simulink model "dds_cwg_1k"  (R2016b)
(part 11 of 84)

      mask help:
      | An explicitly laid-out delay line to avoid mapping to SRL16s
      | for use in pipelining to help achieve timing closure.
      mask init:
      | pipeline_init(gcb,'latency',latency);
      settings: AttributesFormatString=Latency = %<latency>
      mask Display:
      | port_label('input', 1, 'd');
      | port_label('output', 1, 'q');
      | disp(['Z^-', num2str(latency)]);
  pipeline99 : Subsystem  Commented=on  AncestorBlock=casper_library_delays/pipeline  mask(pipeline){latency=2}
      mask help:
      | An explicitly laid-out delay line to avoid mapping to SRL16s
      | for use in pipelining to help achieve timing closure.
      mask init:
      | pipeline_init(gcb,'latency',latency);
      settings: AttributesFormatString=Latency = %<latency>
      mask Display:
      | port_label('input', 1, 'd');
      | port_label('output', 1, 'q');
      | disp(['Z^-', num2str(latency)]);
  pulse_ext : casper_library_misc/pulse_ext  pulse_len=10
  pulse_ext1 : casper_library_misc/pulse_ext  pulse_len=10
  register_change_detect : Subsystem  Commented=on
  ss_fft : Subsystem  Tag=casper:bitsnap  Commented=on  AncestorBlock=casper_library_scopes/bitfield_snapshot  mask(bitsnap){io_names=[re im ch dv sync of], io_widths=[18 18 15 1 1 1], io_bps=[0 0 0 0 0 0], io_types=[0 0 0 2 2 2], show_format=on, snap_storage=bram, snap_dram_dimm=2, snap_dram_clock=250, snap_nsamples=8, snap_data_width=64, snap_offset=on, snap_circap=off, snap_value=off, snap_ext_arm=off, snap_ext_circ=off, snap_provide_outputs=on, snap_use_dsp48=on, snap_delay=0, extra_names=[c d], extra_widths=[30 2], extra_bps=[0 0], extra_types=0}
      mask prompts: io_names "Names [msb...lsb]"; io_widths "Bitwidths [msb...lsb]"; io_bps "Binary pts [msb...lsb]"; io_types "Data types [msb...lsb], ufix=0, fix=1, bool=2"; show_format "Print format string?"; snap_storage "Storage medium"; snap_dram_dimm "DRAM dimm"; snap_dram_clock "DRAM clock rate"; snap_nsamples "Number of Samples (2^?)"; snap_data_width "Data width"; snap_offset "Start delay support"; snap_circap "Circular capture support"; snap_value "Extra value capture support"; snap_ext_arm "External arm support"; snap_ext_circ "External circular capture support"; snap_provide_outputs "Provide outputs"; snap_use_dsp48 "Use DSP48s to implement counters"; snap_delay "Pre-snapshot delay"; extra_names "Names [msb...lsb]"; extra_widths "Widths [msb...lsb]"; extra_bps "Binary pts [msb...lsb]"; extra_types "Data types [msb...lsb], ufix=0, fix=1, bool=2"
      mask help:
      | A wrapped snapshot block. Allows specification of inputs to a snapblock word so the toolflow can automatically set up the scope.
      | See documentation for snapshot for explanation of parameters.
      mask init:
      | bitsnap_init(gcb);
      settings: AttributesFormatString=|
      | snap(6):uf18.0,uf18.0,uf15.0,b,b,b = 54 bits\n64 wide, 256 deep
      | debugID: 24471511
      mask TypeOptions snap_storage: bram | dram
      mask Callback snap_storage: bitsnap_callback();
      mask TypeOptions snap_dram_dimm: 1 | 2 | 3 | 4
      mask TypeOptions snap_dram_clock: 200 | 250 | 266 | 300 | 333
      mask TypeOptions snap_data_width: 8 | 16 | 32 | 64 | 128
      mask Callback snap_value: bitsnap_callback();
      mask Callback snap_ext_arm: bitsnap_callback();
      mask Callback snap_ext_circ: bitsnap_callback();
      mask Callback snap_provide_outputs: bitsnap_callback();
  ss_fft1 : Subsystem  Tag=casper:bitsnap  Commented=on  AncestorBlock=casper_library_scopes/bitfield_snapshot  mask(bitsnap){io_names=[re im ch dv sync], io_widths=[18 18 15 1 1], io_bps=[0 0 0 0 0], io_types=[0 0 0 2 2], show_format=on, snap_storage=bram, snap_dram_dimm=2, snap_dram_clock=250, snap_nsamples=9, snap_data_width=64, snap_offset=on, snap_circap=off, snap_value=off, snap_ext_arm=off, snap_ext_circ=off, snap_provide_outputs=on, snap_use_dsp48=on, snap_delay=0, extra_names=[c d], extra_widths=[30 2], extra_bps=[0 0], extra_types=0}
      mask prompts: io_names "Names [msb...lsb]"; io_widths "Bitwidths [msb...lsb]"; io_bps "Binary pts [msb...lsb]"; io_types "Data types [msb...lsb], ufix=0, fix=1, bool=2"; show_format "Print format string?"; snap_storage "Storage medium"; snap_dram_dimm "DRAM dimm"; snap_dram_clock "DRAM clock rate"; snap_nsamples "Number of Samples (2^?)"; snap_data_width "Data width"; snap_offset "Start delay support"; snap_circap "Circular capture support"; snap_value "Extra value capture support"; snap_ext_arm "External arm support"; snap_ext_circ "External circular capture support"; snap_provide_outputs "Provide outputs"; snap_use_dsp48 "Use DSP48s to implement counters"; snap_delay "Pre-snapshot delay"; extra_names "Names [msb...lsb]"; extra_widths "Widths [msb...lsb]"; extra_bps "Binary pts [msb...lsb]"; extra_types "Data types [msb...lsb], ufix=0, fix=1, bool=2"
      mask help:
      | A wrapped snapshot block. Allows specification of inputs to a snapblock word so the toolflow can automatically set up the scope.
      | See documentation for snapshot for explanation of parameters.
      mask init:
      | bitsnap_init(gcb);
      settings: AttributesFormatString=|
      | snap(5):uf18.0,uf18.0,uf15.0,b,b = 53 bits\n64 wide, 512 deep
      | debugID: 87522550
      mask TypeOptions snap_storage: bram | dram
      mask Callback snap_storage: bitsnap_callback();
      mask TypeOptions snap_dram_dimm: 1 | 2 | 3 | 4
      mask TypeOptions snap_dram_clock: 200 | 250 | 266 | 300 | 333
      mask TypeOptions snap_data_width: 8 | 16 | 32 | 64 | 128
      mask Callback snap_value: bitsnap_callback();
      mask Callback snap_ext_arm: bitsnap_callback();
      mask Callback snap_ext_circ: bitsnap_callback();
      mask Callback snap_provide_outputs: bitsnap_callback();
  ss_fft2 : Subsystem  Tag=casper:bitsnap  Commented=on  AncestorBlock=casper_library_scopes/bitfield_snapshot  mask(bitsnap){io_names=[re im ch dv sync], io_widths=[18 18 15 1 1], io_bps=[0 0 0 0 0], io_types=[0 0 0 2 2], show_format=on, snap_storage=bram, snap_dram_dimm=2, snap_dram_clock=250, snap_nsamples=9, snap_data_width=64, snap_offset=on, snap_circap=off, snap_value=off, snap_ext_arm=off, snap_ext_circ=off, snap_provide_outputs=on, snap_use_dsp48=on, snap_delay=0, extra_names=[c d], extra_widths=[30 2], extra_bps=[0 0], extra_types=0}
      mask prompts: io_names "Names [msb...lsb]"; io_widths "Bitwidths [msb...lsb]"; io_bps "Binary pts [msb...lsb]"; io_types "Data types [msb...lsb], ufix=0, fix=1, bool=2"; show_format "Print format string?"; snap_storage "Storage medium"; snap_dram_dimm "DRAM dimm"; snap_dram_clock "DRAM clock rate"; snap_nsamples "Number of Samples (2^?)"; snap_data_width "Data width"; snap_offset "Start delay support"; snap_circap "Circular capture support"; snap_value "Extra value capture support"; snap_ext_arm "External arm support"; snap_ext_circ "External circular capture support"; snap_provide_outputs "Provide outputs"; snap_use_dsp48 "Use DSP48s to implement counters"; snap_delay "Pre-snapshot delay"; extra_names "Names [msb...lsb]"; extra_widths "Widths [msb...lsb]"; extra_bps "Binary pts [msb...lsb]"; extra_types "Data types [msb...lsb], ufix=0, fix=1, bool=2"
      mask help:
      | A wrapped snapshot block. Allows specification of inputs to a snapblock word so the toolflow can automatically set up the scope.
      | See documentation for snapshot for explanation of parameters.
      mask init:
      | bitsnap_init(gcb);
      settings: AttributesFormatString=|
      | snap(5):uf18.0,uf18.0,uf15.0,b,b = 53 bits\n64 wide, 512 deep
      | debugID: 87552341
      mask TypeOptions snap_storage: bram | dram
      mask Callback snap_storage: bitsnap_callback();
      mask TypeOptions snap_dram_dimm: 1 | 2 | 3 | 4
      mask TypeOptions snap_dram_clock: 200 | 250 | 266 | 300 | 333
      mask TypeOptions snap_data_width: 8 | 16 | 32 | 64 | 128
      mask Callback snap_value: bitsnap_callback();
      mask Callback snap_ext_arm: bitsnap_callback();
      mask Callback snap_ext_circ: bitsnap_callback();
      mask Callback snap_provide_outputs: bitsnap_callback();
  ss_fft3 : Subsystem  Tag=casper:bitsnap  Commented=on  AncestorBlock=casper_library_scopes/bitfield_snapshot  mask(bitsnap){io_names=[re im shift dv_in sync rst tlast dv_out ch0 re_ou sync_out dvu trdy err fifo], io_widths=[18 18 16 1 1 1 1 1 15 18 1 1 1 1 1], io_bps=[0 0 0 0 0 0 0 0 0 0 0 0 0 0 0], io_types=[0 0 0 2 2 2 2 2 0 0 2 2 2 2 2], show_format=on, snap_storage=bram, snap_dram_dimm=2, snap_dram_clock=250, snap_nsamples=10, snap_data_width=128, snap_offset=on, snap_circap=off, snap_value=off, snap_ext_arm=off, snap_ext_circ=off, snap_provide_outputs=on, snap_use_dsp48=on, snap_delay=0, extra_names=[c d], extra_widths=[30 2], extra_bps=[0 0], extra_types=0}
      mask prompts: io_names "Names [msb...lsb]"; io_widths "Bitwidths [msb...lsb]"; io_bps "Binary pts [msb...lsb]"; io_types "Data types [msb...lsb], ufix=0, fix=1, bool=2"; show_format "Print format string?"; snap_storage "Storage medium"; snap_dram_dimm "DRAM dimm"; snap_dram_clock "DRAM clock rate"; snap_nsamples "Number of Samples (2^?)"; snap_data_width "Data width"; snap_offset "Start delay support"; snap_circap "Circular capture support"; snap_value "Extra value capture support"; snap_ext_arm "External arm support"; snap_ext_circ "External circular capture support"; snap_provide_outputs "Provide outputs"; snap_use_dsp48 "Use DSP48s to implement counters"; snap_delay "Pre-snapshot delay"; extra_names "Names [msb...lsb]"; extra_widths "Widths [msb...lsb]"; extra_bps "Binary pts [msb...lsb]"; extra_types "Data types [msb...lsb], ufix=0, fix=1, bool=2"
      mask help:
      | A wrapped snapshot block. Allows specification of inputs to a snapblock word so the toolflow can automatically set up the scope.
      | See documentation for snapshot for explanation of parameters.
      mask init:
      | bitsnap_init(gcb);
      settings: AttributesFormatString=|
      | snap(15):uf18.0,uf18.0,uf16.0,b,b,b,b,b,uf15.0,uf18.0,b,b,b,b,b = 95 bits\n128 wide, 1024 deep
      | debugID: 87582132
      mask TypeOptions snap_storage: bram | dram
      mask Callback snap_storage: bitsnap_callback();
      mask TypeOptions snap_dram_dimm: 1 | 2 | 3 | 4
      mask TypeOptions snap_dram_clock: 200 | 250 | 266 | 300 | 333
      mask TypeOptions snap_data_width: 8 | 16 | 32 | 64 | 128
      mask Callback snap_value: bitsnap_callback();
      mask Callback snap_ext_arm: bitsnap_callback();
      mask Callback snap_ext_circ: bitsnap_callback();
      mask Callback snap_provide_outputs: bitsnap_callback();
  ss_fft4 : Subsystem  Tag=casper:bitsnap  Commented=on  AncestorBlock=casper_library_scopes/bitfield_snapshot  mask(bitsnap){io_names=[re_i re_o dv we rd sync empty full dv_in dcount], io_widths=[18 18 1 1 1 1 1 1 1 6], io_bps=[0 0 0 0 0 0 0 0 0 0], io_types=[0 0 2 2 2 2 2 2 2 0], show_format=on, snap_storage=bram, snap_dram_dimm=2, snap_dram_clock=250, snap_nsamples=10, snap_data_width=64, snap_offset=on, snap_circap=off, snap_value=off, snap_ext_arm=off, snap_ext_circ=off, snap_provide_outputs=on, snap_use_dsp48=on, snap_delay=0, extra_names=[c d], extra_widths=[30 2], extra_bps=[0 0], extra_types=0}
      mask prompts: io_names "Names [msb...lsb]"; io_widths "Bitwidths [msb...lsb]"; io_bps "Binary pts [msb...lsb]"; io_types "Data types [msb...lsb], ufix=0, fix=1, bool=2"; show_format "Print format string?"; snap_storage "Storage medium"; snap_dram_dimm "DRAM dimm"; snap_dram_clock "DRAM clock rate"; snap_nsamples "Number of Samples (2^?)"; snap_data_width "Data width"; snap_offset "Start delay support"; snap_circap "Circular capture support"; snap_value "Extra value capture support"; snap_ext_arm "External arm support"; snap_ext_circ "External circular capture support"; snap_provide_outputs "Provide outputs"; snap_use_dsp48 "Use DSP48s to implement counters"; snap_delay "Pre-snapshot delay"; extra_names "Names [msb...lsb]"; extra_widths "Widths [msb...lsb]"; extra_bps "Binary pts [msb...lsb]"; extra_types "Data types [msb...lsb], ufix=0, fix=1, bool=2"
      mask help:
      | A wrapped snapshot block. Allows specification of inputs to a snapblock word so the toolflow can automatically set up the scope.
      | See documentation for snapshot for explanation of parameters.
      mask init:
      | bitsnap_init(gcb);
      settings: AttributesFormatString=|
      | snap(10):uf18.0,uf18.0,b,b,b,b,b,b,b,uf6.0 = 49 bits\n64 wide, 1024 deep
      | debugID: 87611923
      mask TypeOptions snap_storage: bram | dram
      mask Callback snap_storage: bitsnap_callback();
      mask TypeOptions snap_dram_dimm: 1 | 2 | 3 | 4
      mask TypeOptions snap_dram_clock: 200 | 250 | 266 | 300 | 333
      mask TypeOptions snap_data_width: 8 | 16 | 32 | 64 | 128
      mask Callback snap_value: bitsnap_callback();
      mask Callback snap_ext_arm: bitsnap_callback();
      mask Callback snap_ext_circ: bitsnap_callback();
      mask Callback snap_provide_outputs: bitsnap_callback();
  ss_fifo_db : Subsystem  Tag=casper:bitsnap  Commented=on  AncestorBlock=casper_library_scopes/bitfield_snapshot  mask(bitsnap){io_names=[din we re rst dout empty full dcount], io_widths=[10 1 1 1 10 1 1 5], io_bps=[0 0 0 0 0 0 0 0], io_types=[0 2 2 2 0 2 2 0], show_format=on, snap_storage=bram, snap_dram_dimm=2, snap_dram_clock=250, snap_nsamples=8, snap_data_width=32, snap_offset=on, snap_circap=off, snap_value=off, snap_ext_arm=off, snap_ext_circ=off, snap_provide_outputs=on, snap_use_dsp48=on, snap_delay=0, extra_names=[c d], extra_widths=[30 2], extra_bps=[0 0], extra_types=0}
      mask prompts: io_names "Names [msb...lsb]"; io_widths "Bitwidths [msb...lsb]"; io_bps "Binary pts [msb...lsb]"; io_types "Data types [msb...lsb], ufix=0, fix=1, bool=2"; show_format "Print format string?"; snap_storage "Storage medium"; snap_dram_dimm "DRAM dimm"; snap_dram_clock "DRAM clock rate"; snap_nsamples "Number of Samples (2^?)"; snap_data_width "Data width"; snap_offset "Start delay support"; snap_circap "Circular capture support"; snap_value "Extra value capture support"; snap_ext_arm "External arm support"; snap_ext_circ "External circular capture support"; snap_provide_outputs "Provide outputs"; snap_use_dsp48 "Use DSP48s to implement counters"; snap_delay "Pre-snapshot delay"; extra_names "Names [msb...lsb]"; extra_widths "Widths [msb...lsb]"; extra_bps "Binary pts [msb...lsb]"; extra_types "Data types [msb...lsb], ufix=0, fix=1, bool=2"
      mask help:
      | A wrapped snapshot block. Allows specification of inputs to a snapblock word so the toolflow can automatically set up the scope.
      | See documentation for snapshot for explanation of parameters.
      mask init:
      | bitsnap_init(gcb);
      settings: AttributesFormatString=|
      | snap(8):uf10.0,b,b,b,uf10.0,b,b,uf5.0 = 30 bits\n32 wide, 256 deep
      | debugID: 59001754
      mask TypeOptions snap_storage: bram | dram
      mask Callback snap_storage: bitsnap_callback();
      mask TypeOptions snap_dram_dimm: 1 | 2 | 3 | 4
      mask TypeOptions snap_dram_clock: 200 | 250 | 266 | 300 | 333
      mask TypeOptions snap_data_width: 8 | 16 | 32 | 64 | 128
      mask Callback snap_value: bitsnap_callback();
      mask Callback snap_ext_arm: bitsnap_callback();
      mask Callback snap_ext_circ: bitsnap_callback();
      mask Callback snap_provide_outputs: bitsnap_callback();
  ss_fir_out : Subsystem  Tag=casper:bitsnap  Commented=on  AncestorBlock=casper_library_scopes/bitfield_snapshot  mask(bitsnap){io_names=[fir_re fir_im dv sync], io_widths=[18 18 1 1], io_bps=[0 17 0 0], io_types=[0 1 2 2], show_format=on, snap_storage=bram, snap_dram_dimm=2, snap_dram_clock=250, snap_nsamples=9, snap_data_width=64, snap_offset=on, snap_circap=off, snap_value=off, snap_ext_arm=off, snap_ext_circ=off, snap_provide_outputs=on, snap_use_dsp48=on, snap_delay=0, extra_names=[c d], extra_widths=[30 2], extra_bps=[0 0], extra_types=0}
      mask prompts: io_names "Names [msb...lsb]"; io_widths "Bitwidths [msb...lsb]"; io_bps "Binary pts [msb...lsb]"; io_types "Data types [msb...lsb], ufix=0, fix=1, bool=2"; show_format "Print format string?"; snap_storage "Storage medium"; snap_dram_dimm "DRAM dimm"; snap_dram_clock "DRAM clock rate"; snap_nsamples "Number of Samples (2^?)"; snap_data_width "Data width"; snap_offset "Start delay support"; snap_circap "Circular capture support"; snap_value "Extra value capture support"; snap_ext_arm "External arm support"; snap_ext_circ "External circular capture support"; snap_provide_outputs "Provide outputs"; snap_use_dsp48 "Use DSP48s to implement counters"; snap_delay "Pre-snapshot delay"; extra_names "Names [msb...lsb]"; extra_widths "Widths [msb...lsb]"; extra_bps "Binary pts [msb...lsb]"; extra_types "Data types [msb...lsb], ufix=0, fix=1, bool=2"
      mask help:
      | A wrapped snapshot block. Allows specification of inputs to a snapblock word so the toolflow can automatically set up the scope.
      | See documentation for snapshot for explanation of parameters.
      mask init:
      | bitsnap_init(gcb);
      settings: AttributesFormatString=|
      | snap(4):uf18.0,f18.17,b,b = 38 bits\n64 wide, 512 deep
      | debugID: 133429805
      mask TypeOptions snap_storage: bram | dram
      mask Callback snap_storage: bitsnap_callback();
      mask TypeOptions snap_dram_dimm: 1 | 2 | 3 | 4
      mask TypeOptions snap_dram_clock: 200 | 250 | 266 | 300 | 333
      mask TypeOptions snap_data_width: 8 | 16 | 32 | 64 | 128
      mask Callback snap_value: bitsnap_callback();
      mask Callback snap_ext_arm: bitsnap_callback();
      mask Callback snap_ext_circ: bitsnap_callback();
      mask Callback snap_provide_outputs: bitsnap_callback();
  ss_nb : Subsystem  Tag=casper:bitsnap  Commented=on  AncestorBlock=casper_library_scopes/bitfield_snapshot  mask(bitsnap){io_names=[r0 i0 r1 i1 sync dv sync_cnt new_spec trig ch], io_widths=[18 18 18 18 1 1 4 1 1 15], io_bps=[17 17 17 17 0 0 0 0 0 0], io_types=[1 1 1 1 2 2 0 2 2 0], show_format=on, snap_storage=bram, snap_dram_dimm=2, snap_dram_clock=250, snap_nsamples=9, snap_data_width=128, snap_offset=off, snap_circap=off, snap_value=off, snap_ext_arm=off, snap_ext_circ=off, snap_provide_outputs=on, snap_use_dsp48=on, snap_delay=2, extra_names=timestamp, extra_widths=32, extra_bps=0, extra_types=0}
      mask prompts: io_names "Names [msb...lsb]"; io_widths "Bitwidths [msb...lsb]"; io_bps "Binary pts [msb...lsb]"; io_types "Data types [msb...lsb], ufix=0, fix=1, bool=2"; show_format "Print format string?"; snap_storage "Storage medium"; snap_dram_dimm "DRAM dimm"; snap_dram_clock "DRAM clock rate"; snap_nsamples "Number of Samples (2^?)"; snap_data_width "Data width"; snap_offset "Start delay support"; snap_circap "Circular capture support"; snap_value "Extra value capture support"; snap_ext_arm "External arm support"; snap_ext_circ "External circular capture support"; snap_provide_outputs "Provide outputs"; snap_use_dsp48 "Use DSP48s to implement counters"; snap_delay "Pre-snapshot delay"; extra_names "Names [msb...lsb]"; extra_widths "Widths [msb...lsb]"; extra_bps "Binary pts [msb...lsb]"; extra_types "Data types [msb...lsb], ufix=0, fix=1, bool=2"
      mask help:
      | A wrapped snapshot block. Allows specification of inputs to a snapblock word so the toolflow can automatically set up the scope.
      | See documentation for snapshot for explanation of parameters.
      mask init:
      | bitsnap_init(gcb);
      settings: AttributesFormatString=|
      | snap(10):f18.17,f18.17,f18.17,f18.17,b,b,uf4.0,b,b,uf15.0 = 95 bits\n128 wide, 512 deep
      | debugID: 12323807
      mask TypeOptions snap_storage: bram | dram
      mask Callback snap_storage: bitsnap_callback();
      mask TypeOptions snap_dram_dimm: 1 | 2 | 3 | 4
      mask TypeOptions snap_dram_clock: 200 | 250 | 266 | 300 | 333
      mask TypeOptions snap_data_width: 8 | 16 | 32 | 64 | 128
      mask Callback snap_value: bitsnap_callback();
      mask Callback snap_ext_arm: bitsnap_callback();
      mask Callback snap_ext_circ: bitsnap_callback();
      mask Callback snap_provide_outputs: bitsnap_callback();
  ss_nb1 : Subsystem  Tag=casper:bitsnap  Commented=on  AncestorBlock=casper_library_scopes/bitfield_snapshot  mask(bitsnap){io_names=[r2 i2 r3 i3 sync dv sync_cnt trig trig_time], io_widths=[18 18 18 18 1 1 4 1 48], io_bps=[17 17 17 17 0 0 0 0 0], io_types=[1 1 1 1 2 2 0 2 0], show_format=on, snap_storage=bram, snap_dram_dimm=2, snap_dram_clock=250, snap_nsamples=9, snap_data_width=128, snap_offset=off, snap_circap=off, snap_value=off, snap_ext_arm=off, snap_ext_circ=off, snap_provide_outputs=on, snap_use_dsp48=on, snap_delay=2, extra_names=timestamp, extra_widths=32, extra_bps=0, extra_types=0}
      mask prompts: io_names "Names [msb...lsb]"; io_widths "Bitwidths [msb...lsb]"; io_bps "Binary pts [msb...lsb]"; io_types "Data types [msb...lsb], ufix=0, fix=1, bool=2"; show_format "Print format string?"; snap_storage "Storage medium"; snap_dram_dimm "DRAM dimm"; snap_dram_clock "DRAM clock rate"; snap_nsamples "Number of Samples (2^?)"; snap_data_width "Data width"; snap_offset "Start delay support"; snap_circap "Circular capture support"; snap_value "Extra value capture support"; snap_ext_arm "External arm support"; snap_ext_circ "External circular capture support"; snap_provide_outputs "Provide outputs"; snap_use_dsp48 "Use DSP48s to implement counters"; snap_delay "Pre-snapshot delay"; extra_names "Names [msb...lsb]"; extra_widths "Widths [msb...lsb]"; extra_bps "Binary pts [msb...lsb]"; extra_types "Data types [msb...lsb], ufix=0, fix=1, bool=2"
      mask help:
      | A wrapped snapshot block. Allows specification of inputs to a snapblock word so the toolflow can automatically set up the scope.
      | See documentation for snapshot for explanation of parameters.
      mask init:
      | bitsnap_init(gcb);
      settings: AttributesFormatString=|
      | snap(9):f18.17,f18.17,f18.17,f18.17,b,b,uf4.0,b,uf48.0 = 127 bits\n128 wide, 512 deep
      | debugID: 113596910
      mask TypeOptions snap_storage: bram | dram
      mask Callback snap_storage: bitsnap_callback();
      mask TypeOptions snap_dram_dimm: 1 | 2 | 3 | 4
      mask TypeOptions snap_dram_clock: 200 | 250 | 266 | 300 | 333
      mask TypeOptions snap_data_width: 8 | 16 | 32 | 64 | 128
      mask Callback snap_value: bitsnap_callback();
      mask Callback snap_ext_arm: bitsnap_callback();
      mask Callback snap_ext_circ: bitsnap_callback();
      mask Callback snap_provide_outputs: bitsnap_callback();
  ss_time_trig_nb : Subsystem  Commented=on
  sync_out : Outport
  dv_out : Outport  Port=2
  pol0_out : Outport  Port=3
  pol1_out : Outport  Port=4
  pfb_of : Outport  Port=5
  tag scope: capture_now=global, current_channel=global, data_pol0=global, fft_ch0=global, fft_ch1=global, fft_conf_tready_p0=global, fft_dv0=global, fft_dv1=global, fft_dvalid=global, fft_p0_fifo_full=global, fft_pol0_err=global, fft_pol0_of=global, fft_pol1_err=global, fft_pol1_of=global, fft_sync0=global, fft_sync=global, fft_sync_count=global, fft_tready_p0=global, fir_data_tlast=global, fir_dvalid_pol0=global, fir_pol0=global, fir_sync=global, reord_channel=global, reord_dv=global, reord_mux_sel=global, reord_pol0=global, reord_pol1=global, reord_sync=global
  wires:
  pfb_fir_generic0/2(pol0_out0) -> pipeline18/1(d)
  pfb_fir_generic1/2(pol0_out0) -> pipeline20/1(d)
  pfb_fir_generic0/1(sync_out) -> pipeline17/1(d)
  pfb_fir_generic1/1(sync_out) -> Terminator5/1
  Reinterpret2/1 -> Concat3/1
  Reinterpret3/1 -> Concat3/2
  Concat3/1 -> [data_pol1]
  pol1/1 -> pfb_fir_generic1/2(pol0_in0)
  Gateway Out21/1 -> To Workspace21/1
  bus_expand1/1(msb_out8) -> Gateway Out21/1
  Gateway Out23/1 -> To Workspace23/1
  bus_expand1/2(out7) -> Gateway Out23/1
  Gateway Out24/1 -> To Workspace24/1
  bus_expand1/3(out6) -> Gateway Out24/1
  Gateway Out25/1 -> To Workspace27/1
  bus_expand1/4(out5) -> Gateway Out25/1
  Gateway Out28/1 -> To Workspace25/1
  bus_expand1/5(out4) -> Gateway Out28/1
  Gateway Out29/1 -> To Workspace28/1
  bus_expand1/6(out3) -> Gateway Out29/1
  Gateway Out30/1 -> To Workspace26/1
  bus_expand1/7(out2) -> Gateway Out30/1
  Gateway Out31/1 -> To Workspace29/1
  bus_expand1/8(lsb_out1) -> Gateway Out31/1
  Gateway Out6/1 -> To Workspace6/1
  Gateway Out1/1 -> To Workspace1/1
  Gateway Out9/1 -> To Workspace9/1
  Gateway Out36/1 -> To Workspace36/1
  Gateway Out39/1 -> To Workspace39/1
  [fft_im_pol1] -> Reinterpret3/1
  [fft_re_pol1] -> Reinterpret2/1
  pfb_fir_generic0/3(dvalid) -> pipeline19/1(d)
  pfb_fir_generic1/3(dvalid) -> pipeline21/1(d)
  Counter1/1 -> pipeline81/1(d), pipeline69/1(d)
  pipeline67/1(q) -> ss_nb/5(in_sync)
  pipeline68/1(q) -> ss_nb/6(in_dv)
  pipeline69/1(q) -> ss_nb/7(in_sync_cnt)
  pipeline70/1(q) -> ss_nb/9(in_trig)
  sync/1 -> pfb_fir_generic1/1(sync), pfb_fir_generic0/1(sync), Gateway Out9/1
  Counter3/1 -> Relational4/1, Gateway Out53/1
  Constant9/1 -> Relational4/2
  bus_expand2/1(msb_out8) -> pipeline87/1(d)
  bus_expand2/2(out7) -> pipeline86/1(d)
  bus_expand2/3(out6) -> pipeline85/1(d)
  bus_expand2/4(out5) -> pipeline84/1(d)
  pipeline84/1(q) -> ss_nb/4(in_i1)
  pipeline85/1(q) -> ss_nb/3(in_r1)
  pipeline86/1(q) -> ss_nb/2(in_i0)
  pipeline87/1(q) -> ss_nb/1(in_r0)
  pipeline79/1(q) -> ss_nb1/5(in_sync)
  pipeline80/1(q) -> ss_nb1/6(in_dv)
  pipeline81/1(q) -> ss_nb1/7(in_sync_cnt)
  pipeline82/1(q) -> ss_nb1/8(in_trig)
  pipeline38/1(q) -> ss_nb1/9(in_trig_time)
  bus_expand2/5(out4) -> pipeline91/1(d)
  bus_expand2/6(out3) -> pipeline90/1(d)
  bus_expand2/7(out2) -> pipeline89/1(d)
  bus_expand2/8(lsb_out1) -> pipeline88/1(d)
  dvalid/1 -> pfb_fir_generic1/3(en), pfb_fir_generic0/3(en), Gateway Out36/1
  Gateway Out70/1 -> To Workspace69/1
  Gateway Out71/1 -> To Workspace70/1
  [fft_re_pol0] -> Gateway Out70/1
  [fft_im_pol0] -> Gateway Out71/1
  pol0/1 -> bus_expand14/1(bus_in), pfb_fir_generic0/2(pol0_in0)
  pipeline88/1(q) -> ss_nb1/4(in_i3)
  pipeline89/1(q) -> ss_nb1/3(in_r3)
  pipeline90/1(q) -> ss_nb1/2(in_i2)
  pipeline91/1(q) -> ss_nb1/1(in_r2)
  pipeline42/1(q) -> ss_nb/8(in_new_spec)
  From149/1 -> pipeline42/1(d)
  fft_shift/1 -> [fft_shift]
  Constant2/1 -> Mux3/2
  [fft_dv0] -> Mux3/1
  Mux3/1 -> [fft_re_pol0]
  Constant1/1 -> Mux4/2
  Mux4/1 -> [fft_im_pol0]
  [fft_re_pol0_int] -> Mux3/3
  [fft_im_pol0_int] -> Mux4/3
  [fft_dv0] -> Mux4/1
  pipeline19/1(q) -> [fir_dvalid_pol0], Gateway Out1/1, Counter3/2
  pipeline20/1(q) -> [fir_pol1]
  pipeline21/1(q) -> [fir_dvalid_pol1]
  pipeline18/1(q) -> [fir_pol0]
  From17/1 -> pipeline79/1(d), pipeline67/1(d)
  [cnt_rst] -> pipeline230/1(d)
  Counter12/1 -> fir_sync_cnt/1(out_reg)
  pipeline229/1(q) -> Counter12/2
  pipeline230/1(q) -> Counter12/1
  From90/1 -> Mux6/1
  Mux6/1 -> edge_detect6/1(in)
  From94/1 -> ss_time_trig_nb/2(rst)
  From91/1 -> ss_time_trig_nb/3(arm)
  ss_time_trig_nb/1(trig) -> Mux6/3
  From95/1 -> ss_time_trig_nb/4(trig_time_in)
  From_pfb_d2/1 -> ss_time_trig_nb/1(current_time)
  From96/1 -> Mux6/2
  pipeline28/1(q) -> ss_nb1/10(we)
  pipeline37/1(q) -> ss_nb/11(we)
  ss_time_trig_nb/2(trig_time) -> pipeline38/1(d)
  edge_detect6/1(out) -> pipeline41/1(d), pipeline82/1(d), pipeline40/1(d), pipeline70/1(d)
  Fast Fourier Transform 9.0 1/1 -> pipeline23/1(d)
  pipeline117/1(q) -> [fft_tready_p0]
  pipeline110/1(q) -> [fft_ch0]
  Gateway Out66/1 -> To Workspace65/1
  Gateway Out67/1 -> To Workspace66/1
  Gateway Out72/1 -> To Workspace71/1
  [fft_dv0] -> Gateway Out67/1
  [fft_ch0] -> Gateway Out66/1
  [fft_tready_p0] -> Gateway Out72/1
  Fast Fourier Transform 9.0 1/5 -> pipeline122/1(d)
  Fast Fourier Transform 9.0 1/6 -> pipeline123/1(d)
  Fast Fourier Transform 9.0 1/8 -> pipeline110/1(d), Relational2/1
  Fast Fourier Transform 9.0 1/15 -> Terminator7/1
  Fast Fourier Transform 9.0 1/16 -> Terminator8/1
  Fast Fourier Transform 9.0 1/17 -> Terminator9/1
  pipeline123/1(q) -> [fft_re_pol0_int]
  pipeline122/1(q) -> [fft_im_pol0_int]
  Inverter1/1 -> Gateway Out41/1, Logical9/2, pipeline62/1(d), Fast Fourier Transform 9.0 1/10
  Gateway Out37/1 -> To Workspace37/1
  [fir_sync] -> pulse_ext/1, Delay9/1
  [fft_sync0] -> Gateway Out37/1
  Concat/1 -> [data_pol0]
  Gateway Out34/1 -> To Workspace32/1
  [fft_sync0] -> [fft_sync]
  [current_channel] -> Gateway Out34/1
  [fft_ch0] -> [current_channel]
  [fft_im_pol0] -> Reinterpret1/1
  [fft_re_pol0] -> Reinterpret/1
  [data_pol0] -> bus_expand16/1(bus_in)
  Gateway Out2/1 -> To Workspace2/1
  Gateway Out5/1 -> To Workspace5/1
  [fft_dv0] -> [fft_dvalid]
  [cnt_rst] -> pipeline27/1(d)
  Counter4/1 -> [fft_sync_count], fft_sync_cnt/1(out_reg)
  pipeline1/1(q) -> Counter4/2
  pipeline27/1(q) -> Counter4/1
  [fft_sync] -> pipeline1/1(d)
  From112/1 -> pipeline68/1(d), pipeline28/1(d), pipeline80/1(d), pipeline37/1(d)
  From114/1 -> bus_expand1/1(bus_in), bus_expand2/1(bus_in)
  Gateway Out18/1 -> To Workspace19/1
  Register11/1 -> Delay26/1
  Register10/1 -> Delay25/1
  Register9/1 -> Delay23/1
  Register1/1 -> Delay22/1
  [capture_now] -> Register1/3
  [capture_now] -> Register9/3
  [capture_now] -> Register10/3
  [capture_now] -> Register11/3
  Gateway Out7/1 -> To Workspace7/1
  Delay19/1 -> Register9/1
  Delay20/1 -> Register10/1
  Gateway Out40/1 -> To Workspace40/1
  [reord_channel] -> Delay5/1
  lsb_1/1 -> Logical4/2
  lsb_0/1 -> Logical4/1
  Logical4/1 -> edge_detect2/1(in)
  [reord_dv] -> Delay1/1
  edge_detect2/1(out) -> [capture_now], Gateway Out40/1
  [capture_now] -> Delay10/1
  Delay10/1 -> Gateway Out61/1, Delay32/1
  Delay1/1 -> Logical4/3
  bus_expand5/1(msb_out2) -> Gateway Out46/1
  bus_expand5/2(lsb_out1) -> Gateway Out49/1
  Delay16/1 -> bus_expand5/1(bus_in), Register1/1
  Gateway Out12/1 -> To Workspace12/1
  Gateway Out13/1 -> To Workspace13/1
  bus_expand4/1(msb_out2) -> Gateway Out13/1
  Gateway Out14/1 -> To Workspace14/1
  bus_expand4/2(lsb_out1) -> Gateway Out14/1
  Gateway Out46/1 -> To Workspace45/1
  Gateway Out49/1 -> To Workspace46/1
  Gateway Out61/1 -> To Workspace49/1
  [reord_dv] -> Delay73/1
  Delay5/1 -> Gateway Out11/1, Delay33/1, Gateway Out12/1, lsb_1/1, lsb_0/1
  Delay33/1 -> Delay34/1
  Gateway Out83/1 -> To Workspace85/1
  [reord_sync] -> Delay78/1
  [reord_pol0] -> Delay74/1
  Delay32/1 -> Delay106/1
  Delay34/1 -> Delay105/1
  Gateway Out11/1 -> To Workspace11/1
  Delay42/1 -> [sync_out]
  [sync_out] -> Gateway Out7/1, sync_out/1
  Register4/1 -> Delay57/1
  Register3/1 -> Delay56/1
  Register7/1 -> Delay54/1
  Register2/1 -> Delay53/1
  [capture_now] -> Register2/3
  [capture_now] -> Register7/3
  [capture_now] -> Register3/3
  [capture_now] -> Register4/3
  Delay51/1 -> Register7/1
  Delay52/1 -> Register3/1
  Delay7/1 -> Register2/1
  [reord_sync] -> Delay62/1
  [reord_pol1] -> Delay76/1
  Gateway Out22/1 -> To Workspace22/1
  bus_expand9/1(msb_out2) -> Gateway Out26/1
  bus_expand9/2(lsb_out1) -> Gateway Out38/1
  Gateway Out26/1 -> To Workspace30/1
  Gateway Out38/1 -> To Workspace38/1
  Delay73/1 -> Gateway Out22/1, Delay19/2, Delay20/2, Delay16/2
  Delay74/1 -> bus_expand9/1(bus_in), bus_expand4/1(bus_in), Register11/1, Delay20/1, Delay19/1, Delay16/1
  [reord_dv] -> Delay75/1
  Delay76/1 -> Register4/1, Delay52/1, Delay51/1, Delay7/1
  Delay75/1 -> Delay51/2, Delay52/2, Delay7/2
  [pol0] -> pol0_out/1
  [pol1] -> pol1_out/1
  [nb_dv] -> Gateway Out18/1, dv_out/1
  From79/1 -> Delay84/1
  Inverter2/1 -> Fast Fourier Transform 9.0 2/10, Logical2/2
  Logical7/1 -> Inverter2/1
  Constant7/1 -> Mux9/2
  [fft_dv1] -> Mux9/1
  Mux9/1 -> [fft_re_pol1]
  Constant6/1 -> Mux10/2
  Mux10/1 -> [fft_im_pol1]
  [fft_re_pol1_int] -> Mux9/3
  [fft_im_pol1_int] -> Mux10/3
  [fft_dv1] -> Mux10/1
  Constant12/1 -> Fast Fourier Transform 9.0 1/8
  Constant10/1 -> Fast Fourier Transform 9.0 1/3
  Constant3/1 -> Fast Fourier Transform 9.0 1/2
  Delay78/1 -> Register1/2, Register11/2, Register10/2, Register9/2
  Delay43/1 -> Delay42/1
  Constant13/1 -> Fast Fourier Transform 9.0 2/3
  Delay81/1 -> Fast Fourier Transform 9.0 2/4
  Delay82/1 -> Fast Fourier Transform 9.0 2/5
  Delay83/1 -> Logical2/1
  Logical2/1 -> Fast Fourier Transform 9.0 2/6
  From118/1 -> Delay83/1
  Delay84/1 -> Fast Fourier Transform 9.0 2/7
  Constant8/1 -> Fast Fourier Transform 9.0 2/9
  pipeline124/1(q) -> [fft_dv0]
  edge_detect3/1(out) -> [fft_sync0]
  edge_detect1/1(out) -> Register5/2
  Register5/1 -> edge_detect3/1(in)
  From47/1 -> bus_expand11/1(bus_in)
  Delay62/1 -> Register7/2, Register3/2, Register4/2, Register2/2
  pipeline40/1(q) -> ss_nb/12(trig)
  pipeline41/1(q) -> ss_nb1/11(trig)
  [fir_pol0] -> bus_expand13/1(bus_in)
  Gateway Out4/1 -> To Workspace4/1
  bus_expand13/1(msb_out2) -> Gateway Out4/1
  Gateway Out8/1 -> To Workspace8/1
  bus_expand13/2(lsb_out1) -> Gateway Out8/1
  bus_expand11/2(lsb_out1) -> Delay81/1
  bus_expand11/1(msb_out2) -> Delay82/1
  bus_expand14/1(msb_out2) -> Gateway Out39/1
  Gateway Out35/1 -> To Workspace35/1
  bus_expand14/2(lsb_out1) -> Gateway Out35/1
  [data_pol0] -> Delay88/1, Delay46/1
  Delay24/1 -> Delay4/1
  [fft_sync] -> Gateway Out33/1, Register12/3, Register12/1
  Gateway Out15/1 -> To Workspace15/1
  Gateway Out17/1 -> To Workspace17/1
  Gateway Out20/1 -> To Workspace20/1
  [current_channel] -> Slice2/1, Slice4/1
  Constant17/1 -> AddSub/2
  AddSub/1 -> Delay3/1
  Delay12/1 -> Single Port RAM/2
  Delay18/1 -> Single Port RAM/1, Gateway Out20/1
  Gateway Out47/1 -> To Workspace48/1
  Delay46/1 -> Delay12/1
  Delay47/1 -> Delay18/1
  Delay3/1 -> Delay99/1
  Reinterpret1/1 -> Concat/2
  Reinterpret/1 -> Concat/1
  bus_expand3/2(lsb_out1) -> Gateway Out17/1
  bus_expand3/1(msb_out2) -> Gateway Out15/1
  Gateway Out50/1 -> To Workspace51/1
  Gateway Out51/1 -> To Workspace3/1
  Gateway Out52/1 -> To Workspace16/1
  bus_expand16/1(msb_out2) -> Gateway Out2/1
  bus_expand16/2(lsb_out1) -> Gateway Out5/1
  [fft_dvalid] -> Gateway Out51/1
  [fft_sync] -> Gateway Out52/1
  Gateway Out3/1 -> To Workspace47/1
  Delay55/1 -> Delay49/1
  Gateway Out16/1 -> To Workspace42/1
  [reord_pol0] -> bus_expand3/1(bus_in)
  [reord_channel] -> Gateway Out50/1
  Delay48/1 -> Delay21/1
  [reord_dv] -> Gateway Out3/1
  [reord_sync] -> Gateway Out16/1
  Logical6/1 -> Delay24/1
  [fft_dvalid] -> Logical6/1
  Inverter/1 -> Logical6/2
  Mux1/1 -> [reord_pol0]
  Single Port RAM/1 -> Mux1/2
  Delay92/1 -> Delay45/1, AddSub/1
  [current_channel] -> Delay92/1
  Delay88/1 -> Delay93/1
  Delay93/1 -> Delay94/1
  Delay94/1 -> Mux1/3
  Delay113/1 -> Mux1/1
  Delay4/1 -> Single Port RAM/3, Gateway Out47/1
  Slice4/1 -> Gateway Out55/1, Delay47/1
  Logical8/1 -> Register12/2, Gateway Out43/1, Delay55/1
  Register12/1 -> Gateway Out27/1, Logical8/2
  [fft_dvalid] -> Logical5/1, Delay95/1
  Delay50/1 -> Delay48/1
  Delay95/1 -> Gateway Out58/1, Delay50/1
  [data_pol1] -> Delay91/1, Delay101/1
  [current_channel] -> Slice6/1, Slice3/1
  Slice3/1 -> Delay115/1, Inverter3/1
  Delay65/1 -> Single Port RAM1/1
  Delay87/1 -> Delay90/1
  Delay91/1 -> Delay63/1
  Delay96/1 -> Delay65/1
  Logical10/1 -> Delay87/1
  [fft_dvalid] -> Logical10/1
  Inverter3/1 -> Logical10/2
  Single Port RAM1/1 -> Mux11/2
  Delay101/1 -> Delay103/1
  Delay103/1 -> Delay104/1
  Delay104/1 -> Mux11/3
  Delay117/1 -> Mux11/1
  Delay90/1 -> Single Port RAM1/3
  Slice6/1 -> Delay96/1
  Mux11/1 -> [reord_pol1]
  From136/1 -> Goto/1
  Gateway Out48/1 -> To Workspace53/1
  Gateway Out53/1 -> To Workspace54/1
  edge_detect9/1(out) -> Gateway Out48/1, [fir_data_tlast]
  Relational4/1 -> edge_detect9/1(in)
  pipeline17/1(q) -> edge_detect10/1(in), Counter3/1
  From12/1 -> Delay98/1, Logical7/1
  Delay98/1 -> Logical7/2
  [fir_sync] -> pipeline229/1(d)
  Delay21/1 -> [reord_dv]
  Delay99/1 -> [reord_channel]
  [reord_sync] -> Register6/3, Register6/1
  Register6/1 -> Logical3/1
  Logical3/1 -> Delay43/1, Register6/2
  Delay63/1 -> Single Port RAM1/2
  Gateway Out19/1 -> To Workspace18/1
  Gateway Out27/1 -> To Workspace31/1
  Gateway Out33/1 -> To Workspace34/1
  Gateway Out43/1 -> To Workspace43/1
  Gateway Out55/1 -> To Workspace56/1
  Logical5/1 -> Delay102/1
  Slice2/1 -> Delay111/1, [reord_mux_sel], Inverter/1
  [reord_mux_sel] -> Gateway Out56/1, Logical5/2
  Gateway Out56/1 -> To Workspace57/1
  Delay45/1 -> Delay86/1
  Delay86/1 -> Delay100/1
  Gateway Out57/1 -> To Workspace58/1
  Delay100/1 -> Gateway Out57/1
  Delay102/1 -> Gateway Out19/1, Logical8/1
  Gateway Out58/1 -> To Workspace59/1
  [capture_now] -> Logical3/2
  Delay106/1 -> [nb_dv]
  Delay107/1 -> bus_expand18/1(bus_in), [pol0]
  Delay108/1 -> [pol1]
  Delay49/1 -> Delay110/1
  edge_detect10/1(out) -> [fir_sync], Gateway Out6/1
  From24/1 -> Counter1/2
  From65/1 -> Counter1/1
  Delay110/1 -> [reord_sync]
  pipeline49/1(q) -> ss_nb/10(in_ch)
  Delay105/1 -> [fft_ch_out]
  [fft_ch_out] -> Gateway Out83/1
  From93/1 -> pipeline49/1(d)
  Delay111/1 -> Delay112/1
  Delay112/1 -> Delay113/1
  Delay116/1 -> Delay117/1
  Delay115/1 -> Delay116/1
  Constant/1 -> Relational2/2
  Relational2/1 -> Logical/1
  Logical/1 -> edge_detect1/1(in)
  Delay109/1 -> Logical/2
  Delay9/1 -> Inverter4/1, Register5/1, Register5/3
  Inverter4/1 -> Logical/3
  Fast Fourier Transform 9.0 2/1 -> Terminator1/1
  Fast Fourier Transform 9.0 2/10 -> Terminator12/1
  Fast Fourier Transform 9.0 2/17 -> Terminator4/1
  Fast Fourier Transform 9.0 2/16 -> Terminator3/1
  Fast Fourier Transform 9.0 2/15 -> Terminator2/1
  Fast Fourier Transform 9.0 2/13 -> Terminator11/1
  Fast Fourier Transform 9.0 2/11 -> Terminator13/1
  Fast Fourier Transform 9.0 2/12 -> Terminator21/1
  Fast Fourier Transform 9.0 2/2 -> Terminator14/1
  Fast Fourier Transform 9.0 2/9 -> pipeline50/1(d)
  Fast Fourier Transform 9.0 2/8 -> pipeline12/1(d)
  Fast Fourier Transform 9.0 2/6 -> pipeline48/1(d)
  Fast Fourier Transform 9.0 2/5 -> pipeline44/1(d)
  Constant5/1 -> Fast Fourier Transform 9.0 2/2
  Fast Fourier Transform 9.0 2/3 -> Terminator15/1
  Fast Fourier Transform 9.0 2/4 -> Terminator16/1
  [fft_pol1_of] -> Concat2/2
  [fft_pol0_of] -> Concat2/1
  Concat2/1 -> pfb_of/1
  Constant4/1 -> Fast Fourier Transform 9.0 1/9
  Constant11/1 -> Fast Fourier Transform 9.0 2/8
  Fast Fourier Transform 9.0 1/3 -> Terminator17/1
  Fast Fourier Transform 9.0 1/4 -> Terminator18/1
  Fast Fourier Transform 9.0 1/13 -> Terminator20/1
  Fast Fourier Transform 9.0 1/12 -> Terminator22/1
  Fast Fourier Transform 9.0 1/11 -> Terminator23/1
  Fast Fourier Transform 9.0 1/10 -> Terminator24/1
  pipeline16/1(q) -> [fft_pol0_of]
  From361/1 -> register_change_detect/1(data)
  register_change_detect/1(state_change) -> edge_detect7/1(in)
  edge_detect7/1(out) -> Goto38/1
  Fast Fourier Transform 9.0 1/7 -> Terminator19/1
  Fast Fourier Transform 9.0 1/14 -> pipeline16/1(d)
  Fast Fourier Transform 9.0 2/14 -> pipeline5/1(d)
  Fast Fourier Transform 9.0 2/7 -> Terminator10/1
  Counter2/1 -> fft_shift_change/1(out_reg)
  pipeline3/1(q) -> Counter2/1
  From45/1 -> pipeline3/1(d)
  pipeline22/1(q) -> Counter2/2
  From46/1 -> pipeline22/1(d)
  pipeline23/1(q) -> [fft_conf_tready_p0]
  From109/1 -> Slice/1
  From13/1 -> Slice1/1
  Slice/1 -> Concat4/2
  Constant14/1 -> Concat4/1
  Slice1/1 -> Concat6/2
  Constant15/1 -> Concat6/1
  Concat6/1 -> Fast Fourier Transform 9.0 2/1
  From43/1 -> Mux2/2
  Concat4/1 -> Mux2/3
  Constant27/1 -> fft_shift_sel/1(sim_1)
  fft_shift_sel/1(in_sel) -> Mux2/1
  From50/1 -> pipeline9/1(d), pipeline7/1(d)
  pipeline7/1(q) -> ss_fir_out/3(in_dv)
  pipeline8/1(q) -> ss_fir_out/4(in_sync)
  pipeline9/1(q) -> ss_fir_out/5(we)
  pipeline25/1(q) -> ss_fir_out/6(trig)
  From16/1 -> pipeline25/1(d), pipeline8/1(d)
  bus_expand12/2(lsb_out1) -> pipeline6/1(d)
  bus_expand12/1(msb_out2) -> pipeline10/1(d)
  From44/1 -> bus_expand12/1(bus_in)
  pipeline6/1(q) -> ss_fir_out/2(in_fir_im)
  pipeline10/1(q) -> Reinterpret10/1
  From58/1 -> pipeline36/1(d)
  From67/1 -> pipeline24/1(d)
  From42/1 -> pipeline39/1(d)
  From55/1 -> pipeline4/1(d), pipeline46/1(d)
  From59/1 -> pipeline47/1(d)
  pipeline24/1(q) -> Reinterpret8/1
  pipeline36/1(q) -> Reinterpret9/1
  pipeline39/1(q) -> ss_fft/3(in_ch)
  pipeline46/1(q) -> ss_fft/4(in_dv)
  pipeline47/1(q) -> ss_fft/6(in_of)
  pipeline4/1(q) -> ss_fft/7(we)
  pipeline11/1(q) -> ss_fft/8(trig)
  From66/1 -> pipeline13/1(d), pipeline11/1(d)
  pipeline13/1(q) -> ss_fft/5(in_sync)
  [fft_im_pol0_int] -> [fft_im_pol1_int]
  [fft_re_pol0_int] -> [fft_re_pol1_int]
  [fft_ch0] -> [fft_ch1]
  [fft_dv0] -> [fft_dv1]
  [fft_pol0_of] -> [fft_pol1_of]
  bus_expand8/2(lsb_out1) -> pipeline30/1(d)
  From78/1 -> pipeline33/1(d), pipeline32/1(d)
  pipeline29/1(q) -> Reinterpret6/1
  pipeline30/1(q) -> Reinterpret7/1
  pipeline31/1(q) -> ss_fft1/3(in_ch)
  pipeline33/1(q) -> ss_fft1/4(in_dv)
  pipeline32/1(q) -> ss_fft1/6(we)
  pipeline15/1(q) -> ss_fft1/7(trig)
  From80/1 -> pipeline15/1(d), pipeline26/1(d)
  pipeline26/1(q) -> ss_fft1/5(in_sync)
  bus_expand8/1(msb_out2) -> pipeline29/1(d)
  bus_expand15/2(lsb_out1) -> pipeline51/1(d)
  From82/1 -> pipeline53/1(d), pipeline54/1(d)
  pipeline43/1(q) -> Reinterpret4/1
  pipeline51/1(q) -> Reinterpret5/1
  pipeline52/1(q) -> ss_fft2/3(in_ch)
  pipeline54/1(q) -> ss_fft2/4(in_dv)
  pipeline53/1(q) -> ss_fft2/6(we)
  pipeline34/1(q) -> ss_fft2/7(trig)
  From81/1 -> pipeline35/1(d), pipeline34/1(d)
  pipeline35/1(q) -> ss_fft2/5(in_sync)
  From84/1 -> pipeline52/1(d)
  bus_expand15/1(msb_out2) -> pipeline43/1(d)
  From83/1 -> bus_expand15/1(bus_in)
  Reinterpret4/1 -> ss_fft2/1(in_re)
  Reinterpret5/1 -> ss_fft2/2(in_im)
  Reinterpret6/1 -> ss_fft1/1(in_re)
  Reinterpret7/1 -> ss_fft1/2(in_im)
  Reinterpret8/1 -> ss_fft/1(in_re)
  Reinterpret9/1 -> ss_fft/2(in_im)
  Reinterpret10/1 -> ss_fir_out/1(in_fir_re)
  From77/1 -> bus_expand8/1(bus_in)
  From76/1 -> pipeline31/1(d)
  [fft_shift] -> Fast Fourier Transform 9.0 1/1
  Mux2/1 -> Terminator6/1
  [fft_shift] -> pipeline59/1(d)
  pipeline57/1(q) -> Reinterpret11/1
  pipeline58/1(q) -> Reinterpret12/1
  pipeline60/1(q) -> ss_fft3/16(we)
  pipeline55/1(q) -> ss_fft3/17(trig)
  pipeline56/1(q) -> ss_fft3/5(in_sync)
  Reinterpret11/1 -> ss_fft3/1(in_re)
  Reinterpret12/1 -> ss_fft3/2(in_im)
  pipeline59/1(q) -> ss_fft3/3(in_shift)
  [fir_sync] -> pipeline55/1(d), pipeline56/1(d)
  pipeline62/1(q) -> ss_fft3/6(in_rst)
  pipeline63/1(q) -> ss_fft3/8(in_dv_out)
  pipeline64/1(q) -> ss_fft3/7(in_tlast)
  [fft_dv0] -> pipeline63/1(d)
  pipeline66/1(q) -> ss_fft3/9(in_ch0)
  [fft_ch0] -> pipeline66/1(d)
  [fft_re_pol0_int] -> pipeline65/1(d)
  pipeline65/1(q) -> Reinterpret14/1
  pipeline71/1(q) -> ss_fft3/11(in_sync_out)
  [fft_sync0] -> pipeline71/1(d)
  Fast Fourier Transform 9.0 1/9 -> Logical9/1, pipeline72/1(d)
  pipeline72/1(q) -> ss_fft3/12(in_dvu)
  pipeline61/1(q) -> ss_fft3/4(in_dv_in)
  Logical9/1 -> pipeline124/1(d), Delay109/1
  [fft_tready_p0] -> edge_detect4/1(in)
  Counter6/1 -> fft_tready_cnt0/1(out_reg)
  edge_detect4/1(out) -> pipeline78/1(d)
  pipeline73/1(q) -> Counter6/1
  [cnt_rst] -> pipeline73/1(d)
  pipeline74/1(q) -> ss_fft3/13(in_trdy)
  Fast Fourier Transform 9.0 1/2 -> pipeline74/1(d), pipeline117/1(d), Inverter5/1
  bus_expand6/1(msb_out2) -> Gateway Out10/1, pipeline57/1(d), Fast Fourier Transform 9.0 1/5
  bus_expand6/2(lsb_out1) -> pipeline58/1(d), Fast Fourier Transform 9.0 1/4
  FIFO/1 -> bus_expand6/1(bus_in), bus_expand17/1(bus_in), bus_expand10/1(bus_in)
  [fir_data_tlast] -> Gateway Out42/1, pipeline64/1(d), Fast Fourier Transform 9.0 1/7
  Logical12/1 -> [fft_pol0_err]
  pipeline75/1(q) -> ss_fft3/14(in_err)
  From105/1 -> pipeline75/1(d)
  Inverter5/1 -> Logical12/1
  pipeline78/1(q) -> Counter6/2
  pulse_ext/1 -> Inverter1/1
  Reinterpret14/1 -> ss_fft3/10(in_re_ou)
  Constant16/1 -> [fft_pol1_err]
  FIFO/3 -> [fft_p0_fifo_full], pipeline96/1(d)
  FIFO/2 -> Inverter6/1, pipeline98/1(d)
  pulse_ext1/1 -> Inverter7/1, pipeline76/1(d), pipeline77/1(d), FIFO/4
  Logical1/1 -> pipeline95/1(d), FIFO/2
  Inverter7/1 -> Logical1/2
  Delay2/1 -> pipeline93/1(d), pipeline94/1(d), Logical1/1
  Delay6/1 -> FIFO/1, bus_expand7/1(bus_in)
  pipeline14/1(q) -> ss_fft3/15(in_fifo)
  From56/1 -> pipeline14/1(d)
  pipeline83/1(q) -> Reinterpret13/1
  pipeline92/1(q) -> Reinterpret15/1
  pipeline94/1(q) -> ss_fft4/11(we)
  pipeline76/1(q) -> ss_fft4/12(trig)
  pipeline77/1(q) -> ss_fft4/6(in_sync)
  pipeline96/1(q) -> ss_fft4/8(in_full)
  Reinterpret13/1 -> ss_fft4/1(in_re_i)
  Reinterpret15/1 -> ss_fft4/2(in_re_o)
  pipeline93/1(q) -> ss_fft4/3(in_dv)
  pipeline95/1(q) -> ss_fft4/4(in_we)
  pipeline97/1(q) -> ss_fft4/5(in_rd)
  pipeline98/1(q) -> ss_fft4/7(in_empty)
  bus_expand7/1(msb_out2) -> pipeline83/1(d)
  bus_expand10/1(msb_out2) -> pipeline92/1(d)
  pipeline99/1(q) -> ss_fft4/9(in_dv_in)
  [cnt_rst] -> pipeline104/1(d)
  Counter5/1 -> fifo_of_cnt/1(out_reg)
  pipeline103/1(q) -> Counter5/2
  pipeline104/1(q) -> Counter5/1
  [fft_p0_fifo_full] -> pipeline103/1(d)
  pipeline100/1(q) -> ss_fft4/10(in_dcount)
  FIFO/4 -> pipeline100/1(d)
  pipeline102/1(q) -> ss_fifo_db/10(trig)
  pipeline109/1(q) -> ss_fifo_db/9(we)
  pipeline101/1(q) -> ss_fifo_db/8(in_dcount)
  pipeline114/1(q) -> ss_fifo_db/1(in_din)
  pipeline112/1(q) -> ss_fifo_db/2(in_we)
  pipeline115/1(q) -> ss_fifo_db/3(in_re)
  pipeline105/1(q) -> ss_fifo_db/7(in_full)
  pipeline106/1(q) -> ss_fifo_db/6(in_empty)
  pipeline107/1(q) -> ss_fifo_db/5(in_dout)
  pipeline108/1(q) -> ss_fifo_db/4(in_rst)
  FIFO1/3 -> pipeline105/1(d)
  FIFO1/4 -> pipeline101/1(d)
  FIFO1/2 -> pipeline106/1(d)
  FIFO1/1 -> pipeline107/1(d)
  Counter7/1 -> pipeline114/1(d), FIFO1/1
  From120/1 -> pipeline109/1(d), pipeline112/1(d), FIFO1/2, Counter7/2
  From57/1 -> Counter7/1, pipeline102/1(d), pipeline108/1(d), FIFO1/4
  Constant18/1 -> pipeline115/1(d), FIFO1/3
  [fft_tready_p0] -> Logical13/2, pipeline97/1(d), FIFO/3
  Inverter6/1 -> Logical13/1
  [fir_pol0] -> Delay6/1
  [fir_dvalid_pol0] -> Delay2/1
  [fir_sync] -> pulse_ext1/1
  Gateway Out10/1 -> To Workspace10/1
  Gateway Out32/1 -> To Workspace33/1
  Gateway Out41/1 -> To Workspace41/1
  Gateway Out42/1 -> To Workspace44/1
  Logical13/1 -> Gateway Out44/1, Logical12/2, pipeline99/1(d), Gateway Out32/1, pipeline60/1(d), pipeline61/1(d), Fast Fourier Transform 9.0 1/6
  Gateway Out44/1 -> To Workspace50/1
  Gateway Out45/1 -> To Workspace52/1
  bus_expand17/1(msb_out2) -> Gateway Out45/1
  Gateway Out54/1 -> To Workspace55/1
  bus_expand18/1(msb_out8) -> Gateway Out54/1
  bus_expand18/2(out7) -> Gateway Out59/1
  Gateway Out59/1 -> To Workspace61/1
  Gateway Out60/1 -> To Workspace62/1
  bus_expand18/3(out6) -> Gateway Out60/1
  Gateway Out62/1 -> To Workspace63/1
  bus_expand18/4(out5) -> Gateway Out62/1
  Gateway Out63/1 -> To Workspace64/1
  bus_expand18/5(out4) -> Gateway Out63/1
  Gateway Out64/1 -> To Workspace67/1
  bus_expand18/6(out3) -> Gateway Out64/1
  Gateway Out65/1 -> To Workspace68/1
  bus_expand18/7(out2) -> Gateway Out65/1
  Gateway Out68/1 -> To Workspace72/1
  bus_expand18/8(lsb_out1) -> Gateway Out68/1
  Concat5/1 -> Delay107/1
  Concat1/1 -> Delay108/1
  Delay22/1 -> Concat5/1
  Delay23/1 -> Concat5/2
  Delay25/1 -> Concat5/3
  Delay26/1 -> Concat5/4
  Delay53/1 -> Concat1/1
  Delay54/1 -> Concat1/2
  Delay56/1 -> Concat1/3
  Delay57/1 -> Concat1/4
